simulink model "phase1"  (R2012b)
settings: Solver=ode45  StartTime=0.0  StopTime=10.0  RelTol=1e-3
settings Model: Creator=zahra  LastModifiedBy=zahra

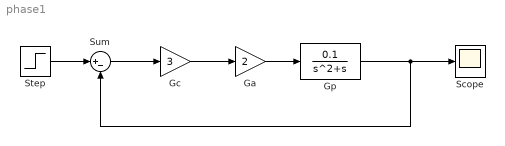
== system phase1 ==
  Ga : Gain  Gain=2
  Gc : Gain  Gain=3
  Gp : TransferFcn  Numerator=[0.1]  Denominator=[1 1 0]
  Scope : Scope
  Step : Step  SampleTime=0
  Sum : Sum  Inputs=|+-
  wires:
  Step/1 -> Sum/1
  Sum/1 -> Gc/1
  Gc/1 -> Ga/1
  Ga/1 -> Gp/1
  Gp/1 -> Sum/2, Scope/1
